simulink model "servo1"  (R2019a)
settings: Solver=VariableStepAuto  StartTime=0.0  StopTime=18.0  RelTol=1e-3
values from neighbouring files (symbols this model uses):
  C = C(1:3,:)    [servo.m]
  K = real(inv(R)*Bbar'*P)    [servo.m]
undefined symbols (not defined in the file or in its folder): A, B, x0, ysp
settings Model: Creator=0210s  LastModifiedBy=0210s

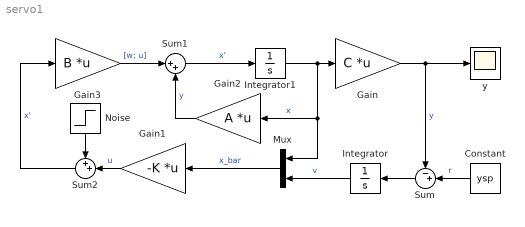
== system servo1 ==
  Constant : Constant  Value=ysp
  Gain : Gain  Gain=C  Multiplication=Matrix(K*u) (u vector)
  Gain1 : Gain  Gain=-K  Multiplication=Matrix(K*u) (u vector)
  Gain2 : Gain  Gain=A  Multiplication=Matrix(K*u) (u vector)
  Gain3 : Gain  Gain=B  Multiplication=Matrix(K*u) (u vector)
  Integrator : Integrator
  Integrator1 : Integrator  InitialCondition=x0
  Mux : Mux  Inputs=2
  Noise : Step  Time=10  Before=[0 0]  After=[-1 1]  SampleTime=0  VectorParams1D=off
  Sum : Sum  Inputs=-+|
  Sum1 : Sum  Inputs=|++
  Sum2 : Sum  Inputs=++|
  y : Scope
  wires:
  Integrator/1 -> Mux/2  "v"
  Sum/1 -> Integrator/1
  Constant/1 -> Sum/2  "r"
  Gain/1 -> y/1, Sum/1  "y"
  Mux/1 -> Gain1/1  "x_bar"
  Integrator1/1 -> Gain2/1, Mux/1, Gain/1  "x"
  Gain2/1 -> Sum1/2  "y"
  Sum1/1 -> Integrator1/1  "x'"
  Gain3/1 -> Sum1/1  "[w; u]"
  Gain1/1 -> Sum2/2  "u"
  Noise/1 -> Sum2/1
  Sum2/1 -> Gain3/1  "x'"
